simulink model "three_phase_THI"  (R2023a)
settings: Solver=daessc  StartTime=0.0  StopTime=.1  MaxStep=1e-4  RelTol=1e-3
libraries: spsIGBTDiodeLib x6, simulink x3, spsSeriesRLCBranchLib x3, spsDCVoltageSourceLib x1, spsVoltageMeasurementLib x1, spspowerguiLib x1
settings Model: Creator=Blu-Ray  LastModifiedBy=Blu-Ray

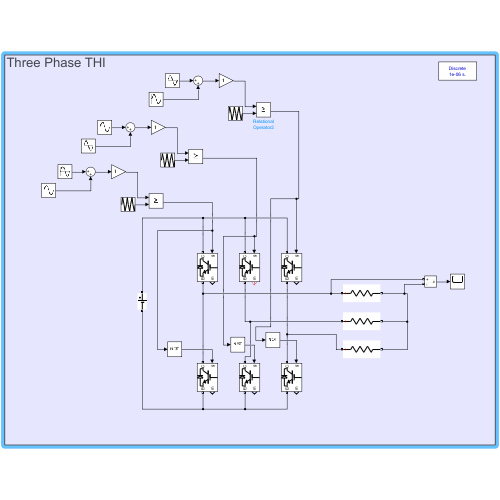
[thumbnail: Simulink's stored preview of the top-level diagram]
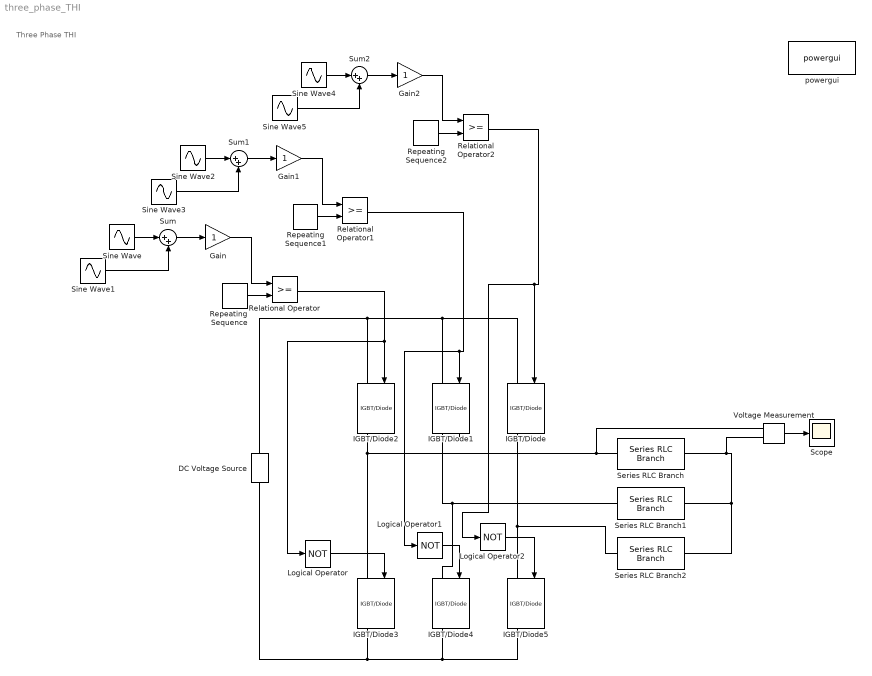
== system three_phase_THI ==
  note: Three Phase THI
  DC Voltage Source : spsDCVoltageSourceLib/DC Voltage Source  Amplitude=300  Measurements=None
  Gain : Gain
  Gain1 : Gain
  Gain2 : Gain
  IGBT/Diode{,1..5} (6 alike) : spsIGBTDiodeLib/IGBT//Diode  Ron=1e-3  Rs=1e5  Cs=inf  Measurements=on
  Logical Operator : Logic  Operator=NOT  AllPortsSameDT=off  OutDataTypeStr=boolean
  Logical Operator1 : Logic  Operator=NOT  AllPortsSameDT=off  OutDataTypeStr=boolean
  Logical Operator2 : Logic  Operator=NOT  AllPortsSameDT=off  OutDataTypeStr=boolean
  Relational Operator : RelationalOperator  OutDataTypeStr=boolean  RndMeth=Simplest  InputSameDT=off
  Relational Operator1 : RelationalOperator  OutDataTypeStr=boolean  RndMeth=Simplest  InputSameDT=off
  Relational Operator2 : RelationalOperator  OutDataTypeStr=boolean  RndMeth=Simplest  InputSameDT=off
  Repeating Sequence : simulink/Sources/Repeating Sequence  rep_seq_t=[0 .25/5000 .5/5000 .75/5000 1/5000]  rep_seq_y=[0 1 0 -1 0]
  Repeating Sequence1 : simulink/Sources/Repeating Sequence  rep_seq_t=[0 .25/5000 .5/5000 .75/5000 1/5000]  rep_seq_y=[0 1 0 -1 0]
  Repeating Sequence2 : simulink/Sources/Repeating Sequence  rep_seq_t=[0 .25/5000 .5/5000 .75/5000 1/5000]  rep_seq_y=[0 1 0 -1 0]
  Scope : Scope
  Series RLC Branch : spsSeriesRLCBranchLib/Series RLC Branch  LConnTagsString=__new0  RConnTagsString=__new0  BranchType=R  Resistance=10  Inductance=1e-3  SetiL0=off  InitialCurrent=0  Capacitance=1e-6  Setx0=off  InitialVoltage=0  Measurements=None
  Series RLC Branch1 : spsSeriesRLCBranchLib/Series RLC Branch  LConnTagsString=__new0  RConnTagsString=__new0  BranchType=R  Resistance=10  Inductance=1e-3  SetiL0=off  InitialCurrent=0  Capacitance=1e-6  Setx0=off  InitialVoltage=0  Measurements=None
  Series RLC Branch2 : spsSeriesRLCBranchLib/Series RLC Branch  LConnTagsString=__new0  RConnTagsString=__new0  BranchType=R  Resistance=10  Inductance=1e-3  SetiL0=off  InitialCurrent=0  Capacitance=1e-6  Setx0=off  InitialVoltage=0  Measurements=None
  Sine Wave : Sin  Amplitude=1.15  Frequency=100*pi  SampleTime=0
  Sine Wave1 : Sin  Amplitude=.19  Frequency=300*pi  SampleTime=0
  Sine Wave2 : Sin  Amplitude=1.15  Frequency=100*pi  Phase=2*pi/3  SampleTime=0
  Sine Wave3 : Sin  Amplitude=.19  Frequency=300*pi  SampleTime=0
  Sine Wave4 : Sin  Amplitude=1.15  Frequency=100*pi  Phase=4*pi/3  SampleTime=0
  Sine Wave5 : Sin  Amplitude=.19  Frequency=300*pi  SampleTime=0
  Sum : Sum  Inputs=|++
  Sum1 : Sum  Inputs=|++
  Sum2 : Sum  Inputs=|++
  Voltage Measurement : spsVoltageMeasurementLib/Voltage Measurement  PhasorSimulation=off  OutputType=Complex  PSBequivalent=0
  powergui : spspowerguiLib/powergui  Priority=1  SimulationMode=Discrete  SampleTime=1e-6  frequency=60  Iterations=50  frequencyindice=0  Pbase=100e6  ErrMax=1e-4  UnitsV=kV  UnitsW=MW  buscounter=0  FunctionMessages=off  echomessages=off  EnableUseOfTLC=off  CurrentSourceSwitches=off  DisableSnubberDevices=off  DisableRonSwitches=off  DisableVfSwitches=off  DisplayEquations=off  AutomaticDiscreteSolvers=off  SolverType=Tustin/Backward Euler (TBE)  Interpol=off  ExternalGateDelay=off  methode=off  Ts=100  x0status=blocks  SPID=on  SwTol=0  HookPort=off  NonlinearTolerance=1e-4  nMaxIteration=100  ContinueOnMaxIteration=off  RestoreLinks=warning  ResistiveCurrentMeasurement=off  Frange=[0:2:500]  Ylog=off  Xlog=on  ShowGrid=off  save=off  variable=ZData  structure=0  ZoomFFT=off  StartTime=0.0  cycles=1  DisplayStyle=1  fundamental=60  FreqAxis=off  MaxFrequency=1000  frequencyindicesteady=1  RmsSteady=1  display=off
  wires:
  Voltage Measurement/1 -> Scope/1
  Sine Wave/1 -> Sum/1
  Sine Wave1/1 -> Sum/2
  Sum/1 -> Gain/1
  Repeating Sequence/1 -> Relational Operator/2
  Gain/1 -> Relational Operator/1
  Relational Operator/1 -> Logical Operator/1, IGBT/Diode2/1
  Logical Operator/1 -> IGBT/Diode3/1
  Relational Operator1/1 -> Logical Operator1/1, IGBT/Diode1/1
  Gain1/1 -> Relational Operator1/1
  Repeating Sequence1/1 -> Relational Operator1/2
  Sum1/1 -> Gain1/1
  Sine Wave3/1 -> Sum1/2
  Sine Wave2/1 -> Sum1/1
  IGBT/Diode1/1 -> ?
  Logical Operator1/1 -> IGBT/Diode4/1
  Sine Wave4/1 -> Sum2/1
  Sine Wave5/1 -> Sum2/2
  Sum2/1 -> Gain2/1
  Repeating Sequence2/1 -> Relational Operator2/2
  Gain2/1 -> Relational Operator2/1
  Relational Operator2/1 -> Logical Operator2/1, IGBT/Diode/1
  Logical Operator2/1 -> IGBT/Diode5/1
  connections:
  IGBT/Diode4/LConn1 -- IGBT/Diode1/RConn1 -- Series RLC Branch1/LConn1
  IGBT/Diode2/RConn1 -- Voltage Measurement/LConn1 -- Series RLC Branch/LConn1 -- IGBT/Diode3/LConn1
  IGBT/Diode/RConn1 -- IGBT/Diode5/LConn1 -- Series RLC Branch2/LConn1
  DC Voltage Source/RConn1 -- IGBT/Diode1/LConn1 -- IGBT/Diode/LConn1 -- IGBT/Diode2/LConn1
  IGBT/Diode5/RConn1 -- IGBT/Diode4/RConn1 -- DC Voltage Source/LConn1 -- IGBT/Diode3/RConn1
  Series RLC Branch/RConn1 -- Voltage Measurement/LConn2 -- Series RLC Branch1/RConn1 -- Series RLC Branch2/RConn1
